simulink model "Galvo_sys_cc_neu_v30"  (R2013a)
settings: Solver=ode45  StartTime=0.0  StopTime=5e-3  MaxStep=1e-4  RelTol=1e-3
InitFcn:
  | Kp_cc = evalin('base','Kp_cc');
  | init = evalin('base','init');
StartFcn:
  | Kp_cc = evalin('base','Kp_cc')
model workspace (MATLAB code in the model file):
  | Kp_cc = evalin('base','Kp_cc');
libraries: simulink x1
settings Model: Kp_cc=1  BufferReuse=off  Creator=mainster  LastModifiedBy=mainster
settings DataIOCC: SaveFormat=StructureWithTime  SignalLoggingSaveFormat=ModelDataLogs
settings OptimizationCC: BlockReduction=off  InlineParams=on  OptimizeBlockIOStorage=off  BufferReuse=off  ExpressionFolding=off  LocalBlockOutputs=off
settings DebuggingCC: MultiTaskDSMMsg=warning  MultiTaskCondExecSysMsg=none  InitInArrayFormatMsg=none  StrictBusMsg=None
settings RTWCC: IncludeERTFirstTime=on
settings GRTTargetCC: CodeReplacementLibrary=None  CPPClassGenCompliant=on

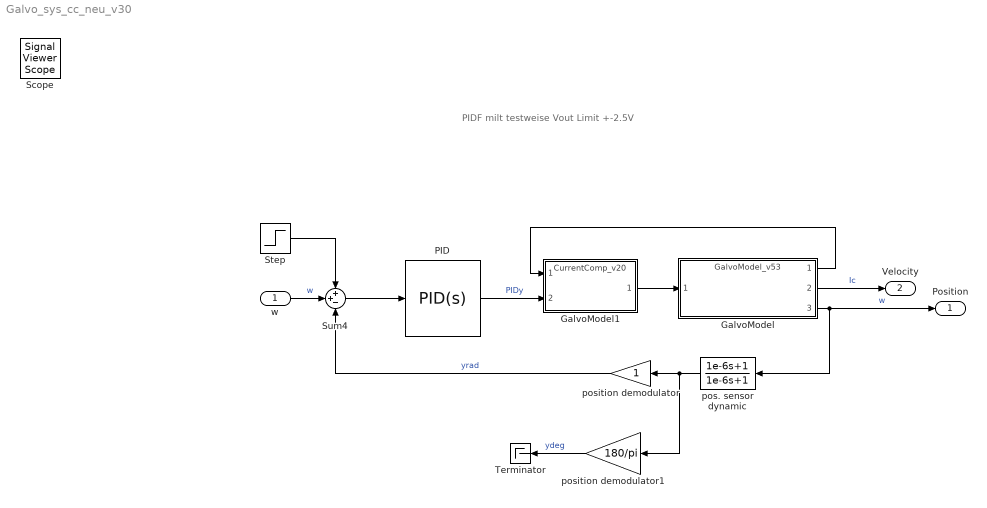
== system Galvo_sys_cc_neu_v30 ==
  note: PIDF milt testweise Vout Limit +-2.5V
  w : Inport
  GalvoModel : ModelReference  ModelNameDialog=GalvoModel_v53.slx  Variant=on  OverrideUsingVariant=v53_neuer_cc  ModelReferenceVersion=1.56  CopyOfModelName=GalvoModel_v53.slx  DefaultDataLogging=on
      mask Display:
      | str=sprintf('%s',get(gcbh,'ModelName'));
      | port_label('input', 1, 'I_{Coil}','texmode','on')
      | color('blue');
      | port_label('output', 3, 'Pos','texmode','on')
      | color('black');
      | port_label('output', 2, 'Speed','texmode','on')
      | port_label('output', 1, 'U_{BEM}','texmode','on')
      | %text(.05,.98,['{\fontsize{12}\it\bf' strrep(str,'_',' ') '}'],'horizontalAlignment','left','verticalAlignment','top','texmode','on')
      | text(.015,.98,['{\fontsize{12}\it\bf' strrep(str,'_','\_') '}'],'horizontalAlignment','left','verticalAlignment','top','texmode','on')
      | text(.15,.05,['{\fontsize{10}\itmechanics}'],'horizontalAlignment','left','verticalAlignment','bottom','texmode','on')
  GalvoModel1 : ModelReference  ModelNameDialog=CurrentComp_v20.slx  Variant=on  OverrideUsingVariant=cc_v20  ModelReferenceVersion=1.60  CopyOfModelName=CurrentComp_v20.slx  DefaultDataLogging=on
      mask Display:
      | str=sprintf('%s',get(gcbh,'ModelName'));
      | port_label('input', 2, 'I_{Set Coil}','texmode','on')
      | color('red');
      | port_label('input', 1, 'U_{BEM}','texmode','on')
      | color('black');
      | port_label('output', 1, 'I_{Coil}','texmode','on')
      | %text(.05,.98,['{\fontsize{12}\it\bf' strrep(str,'_',' ') '}'],'horizontalAlignment','left','verticalAlignment','top','texmode','on')
      | text(.95,0.95,['{\fontsize{12}\it\bfG_{cc}(s)}'],'horizontalAlignment','right','verticalAlignment','top','texmode','on')
      | %text(.15,.05,['{\fontsize{10}\itmechanics}'],'horizontalAlignment','left','verticalAlignment','bottom','texmode','on')
  PID : simulink/Continuous/PID Controller  Controller=PID  TimeDomain=Continuous-time  SampleTime=1  IntegratorMethod=Forward Euler  FilterMethod=Forward Euler  Form=Ideal  P=22.6304684101846  I=17.1701026929863  D=0.000767663019594148*1  N=7253.10376400166  InitialConditionSource=internal  InitialConditionForIntegrator=0  InitialConditionForFilter=0  ExternalReset=none  IgnoreLimit=on  LimitOutput=off  UpperSaturationLimit=25  LowerSaturationLimit=-25  LinearizeAsGain=off  AntiWindupMode=clamping  Kb=6  TrackingMode=off  Kt=0  PParamMin=[]  PParamMax=[]  IParamMin=[]  IParamMax=[]  DParamMin=[]  DParamMax=[]  NParamMin=[]  NParamMax=[]  KbParamMin=[]  KbParamMax=[]  KtParamMin=[]  KtParamMax=[]  POutMin=[]  POutMax=[]  IOutMin=[]  IOutMax=[]  DOutMin=[]  DOutMax=[]  NOutMin=[]  NOutMax=[]  KbOutMin=[]  KbOutMax=[]  KtOutMin=[]  KtOutMax=[]  IntegratorOutMin=[]  IntegratorOutMax=[]  FilterOutMin=[]  FilterOutMax=[]  SumOutMin=[]  SumOutMax=[]  SumI1OutMin=[]  SumI1OutMax=[]  SumI2OutMin=[]  SumI2OutMax=[]  SumI3OutMin=[]  SumI3OutMax=[]  SumDOutMin=[]  SumDOutMax=[]  SaturationOutMin=[]  SaturationOutMax=[]  IntegratorContinuousStateAttributes=''  IntegratorStateMustResolveToSignalObject=off  IntegratorRTWStateStorageClass=Auto  FilterContinuousStateAttributes=''  FilterStateMustResolveToSignalObject=off  FilterRTWStateStorageClass=Auto
      settings: AttributesFormatString=AWM=%<AntiWindupMode>\nD=%<D>\nI=%<I>\nN=%<N>\nP=%<P>\nLimit=+-%<UpperSaturationLimit>
  Step : Step  Time=1e-3  After=0.2  SampleTime=0  ZeroCross=off
      settings: AttributesFormatString=Ampl.: %<After>
  Sum4 : Sum  Inputs=++-
  Terminator : Terminator
  pos. sensor dynamic : TransferFcn  Numerator=[1e-6 1]  Denominator=[1e-6 1]
  position demodulator : Gain
  position demodulator1 : Gain  Gain=180/pi
  Position : Outport
  Velocity : Outport  Port=2
  Scope : SignalViewerScope  IOType=viewer  RefreshTime=0.035000
  wires:
  Sum4/1 -> PID/1
  Step/1 -> Sum4/1
  w/1 -> Sum4/2  "w"
  pos. sensor dynamic/1 -> position demodulator1/1, position demodulator/1
  position demodulator1/1 -> Terminator/1  "ydeg"
  position demodulator/1 -> Sum4/3  "yrad"
  GalvoModel1/1 -> GalvoModel/1
  GalvoModel/2 -> Velocity/1  "Ic"
  GalvoModel/3 -> pos. sensor dynamic/1, Position/1  "w"
  PID/1 -> GalvoModel1/2  "PIDy"
  GalvoModel/1 -> GalvoModel1/1
